simulink model "vipliveedgedetection_win"  (R2022b)
settings: Solver=FixedStepDiscrete  StartTime=0.0  StopTime=inf  RelTol=1e-3  EnableMultiTasking=on
undefined symbols (not defined in the file or in its folder): EdgeTrigger, FallingEdge, gray, videoinput
libraries: visiontextngfix x1, visionanalysis x1, imaqlib x1, vipmisc x1
settings Model: FPTRunName=Active  Creator=The MathWorks, Inc.  LastModifiedBy=The MathWorks, Inc.
settings SolverCC: AlgebraicLoopSolver=TrustRegion
settings DataIOCC: SaveFormat=Array  SaveOutput=off  SaveTime=off  ReturnWorkspaceOutputs=off  SignalLoggingName=sigsOut
settings OptimizationCC: ExpressionDepthLimit=2147483647  InitFltsAndDblsToZero=on  LifeSpan=inf
settings DebuggingCC: UnderspecifiedInitializationDetection=Classic  MergeDetectMultiDrivingBlocksExec=none  CheckExecutionContextPreStartOutputMsg=on  SignalResolutionControl=TryResolveAllWithWarning  MultiTaskDSMMsg=warning  MultiTaskCondExecSysMsg=none  SigSpecEnsureSampleTimeMsg=none  FcnCallInpInsideContextMsg=warning  UnconnectedInputMsg=warning  UnconnectedOutputMsg=warning  UnconnectedLineMsg=warning  StateNameClashWarn=warning  SFUnexpectedBacktrackingDiag=warning  SFNoUnconditionalDefaultTransitionDiag=warning  SFExecutionAtInitializationDiag=none  SFMachineParentedDataDiag=warning  ArithmeticOperatorsInVariantConditions=warning
settings HardwareCC: ProdBitPerPointer=32  ProdBitPerSizeT=32  ProdBitPerPtrDiffT=32  ProdLargestAtomicFloat=None  ProdIntDivRoundTo=Undefined  ProdEndianess=Unspecified  ProdWordSize=32  ProdHWDeviceType=32-bit Generic  TargetBitPerLong=64  TargetBitPerPointer=64  TargetBitPerSizeT=64  TargetBitPerPtrDiffT=64  TargetLongLongMode=on  TargetIntDivRoundTo=Zero  TargetEndianess=LittleEndian  TargetWordSize=64  TargetHWDeviceType=Generic->MATLAB Host Computer  ProdEqTarget=off
settings ModelReferenceCC: EnableRefExpFcnMdlSchedulingChecks=on  PropagateSignalLabelsOutOfModel=off
settings SFSimCC: SimUseLocalCustomCode=off  CustomCodeUndefinedFunction=UseInterfaceOnly
settings RTWCC: RTWUseLocalCustomCode=off
settings CodeAppCC: StateflowObjectComments=on
settings GRTTargetCC: TargetFcnLib=ansi_tfl_tmw_new.mat  TargetLangStandard=C89/C90 (ANSI)  CombineOutputUpdateFcns=off  GRTInterface=on
settings ConfigComp: CovMetricSettings=dw  CovSaveCumulativeToWorkspaceVar=on  CovSaveSingleToWorkspaceVar=on  CovExternalEMLEnable=off

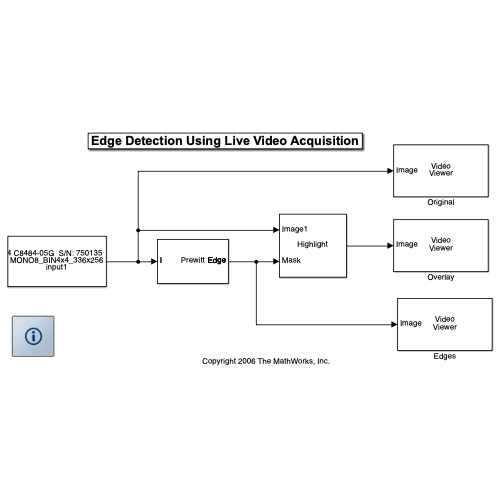
[thumbnail: Simulink's stored preview of the top-level diagram]
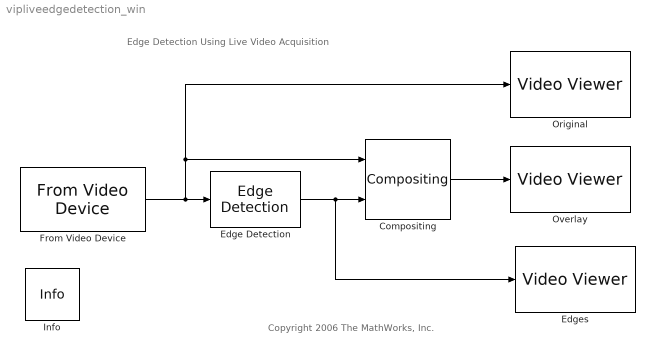
== system vipliveedgedetection_win ==
  note: Edge Detection Using Live Video Acquisition
  note: Copyright 2006 The MathWorks, Inc.
  Compositing : visiontextngfix/Compositing  operation=Highlight selected pixels  bFacSrc=Input port  bFactor=0.75  mFacSrc=Input port  mFactor=1  source=Specify via dialog  coordinates=[1 1]  roundingMode=Floor  overflowMode=off  prodOutputMode=Binary point scaling  prodOutputWordLength=32  prodOutputFracLength=10
  Edge Detection : visionanalysis/Edge Detection  method=Prewitt  outputType=Binary image  userDefinedThreshold=on  thresholdSource=Specify via dialog  threshold=single(15/256)  thresholdTuning=4  edgeThinning=on  threshold_canny=[0.25 0.60]  autoPercent=70  sigma=1  roundingMode=Floor  overflowMode=off
  Edges : VideoViewer  colormapValue=gray(256)  FigPos=[517 473 343 299]  trueSizedOnce=on
  From Video Device : imaqlib/From Video Device  DeviceMenu=demo 1 (Color Device)  Device="hamamatsu 1 (Hamamatsu 1394 C8484-05G  S/N: 750135  Bus: OHCI 1394)"  ObjConstructor=videoinput('hamamatsu', 1)  VideoFormatMenu=RGB_NTSC  VideoFormat=MONO8_BIN4x4_336x256  VideoSource=input1  ROIPosition=[0 0 256 336]  EnableHWTrigger=off  TriggerConfiguration=EdgeTrigger/FallingEdge  SampleTime=1/30  OutputPortsMode=One multidimensional signal  DataType=single  CanDoHWTrigger=yes  ReturnedColorSpace=grayscale  BlockHandle=30.1971  ROIWidth=336  ROIHeight=256  ROIColumn=0  ROIRow=0  EngXMLPath=/System/Volumes/Data/mathworks/devel/bat/filer/batfs2510-0/BR2022bd.2041392.BR2022bd.2041231.pass/build/matlab/toolbox/imaq/imaq/private  DevXMLPath=/mathworks/devel/sandbox/wjachimc/Adsp/matlab/toolbox/imaq/imaqadaptors/glnxa64  EngLibPath=/System/Volumes/Data/mathworks/devel/bat/filer/batfs2510-0/BR2022bd.2041392.BR2022bd.2041231.pass/build/matlab/toolbox/imaq/imaqblks/imaqmex/maci64  ColorSpace=rgb  BayerSensorAlignment=grbg  ImaqMode=off
  Info : vipmisc/Info  SystemSampleTime=-1  VariantActivationTime=update diagram  Latency=0  AutoFrameSizeCalculation=off
  Original : VideoViewer  colormapValue=gray(256)  FigPos=[78 476 363 305]  trueSizedOnce=on
  Overlay : VideoViewer  colormapValue=gray(256)  FigPos=[306 474 353 302]  trueSizedOnce=on
  wires:
  From Video Device/1 -> Edge Detection/1, Original/1, Compositing/1
  Compositing/1 -> Overlay/1
  Edge Detection/1 -> Edges/1, Compositing/2
